simulink model "FOC"  (R2023b)
settings: Solver=FixedStepAuto  StartTime=0.0  StopTime=10.0  FixedStep=1e-4  RelTol=1e-3
settings Model: DataDictionary=FOC.sldd  Creator=18575  LastModifiedBy=18575
settings OptimizationCC: DefaultParameterBehavior=Inlined  UseDivisionForNetSlopeComputation=on  GainParamInheritBuiltInType=on  UseFloatMulNetSlope=on  InlineInvariantSignals=on  PassReuseOutputArgsAs=Individual arguments  ZeroExternalMemoryAtStartup=off  ZeroInternalMemoryAtStartup=off  NoFixptDivByZeroProtection=on  EfficientFloat2IntCast=on  LifeSpan=1  OptimizeBlockOrder=speed  DifferentSizesBufferReuse=on  EfficientTunableParamExpr=on
settings DebuggingCC: ParameterTunabilityLossMsg=error
settings HardwareCC: ProdBitPerPointer=32  ProdBitPerSizeT=32  ProdBitPerPtrDiffT=32  ProdLargestAtomicInteger=Long  ProdLargestAtomicFloat=Double  ProdWordSize=32  ProdLongLongMode=on  ProdHWDeviceType=ARM Compatible->ARM Cortex-M
settings SFSimCC: MATLABDynamicMemAlloc=off
settings RTWCC: Description=Embedded Coder  SystemTargetFile=ert.tlc  TemplateMakefile=ert_default_tmf  GenerateReport=on  LaunchReport=on
settings CodeAppCC: ForceParamTrailComments=on  IgnoreCustomStorageClasses=off  OperatorAnnotations=on  SimulinkDataObjDesc=on  SFDataObjDesc=on  CustomSymbolStrGlobalVar=rt$N$M  CustomSymbolStrType=$N$M  CustomSymbolStrFcn=$N$M$F  CustomSymbolStrMacro=$N$M  InsertBlockDesc=on
settings ERTTargetCC: TargetLangStandard=C99 (ISO)  CodeReplacementLibrary=ARM Cortex-M  GenerateSampleERTMain=on  IncludeMdlTerminateFcn=off  CombineSignalStateStructs=on  SuppressErrorStatus=on  SupportAbsoluteTime=off  SupportNonFinite=off  SupportComplex=off  InlinedParameterPlacement=NonHierarchical  ERTCustomFileTemplate=example_file_process.tlc  ERTFilePackagingFormat=CompactWithDataFile

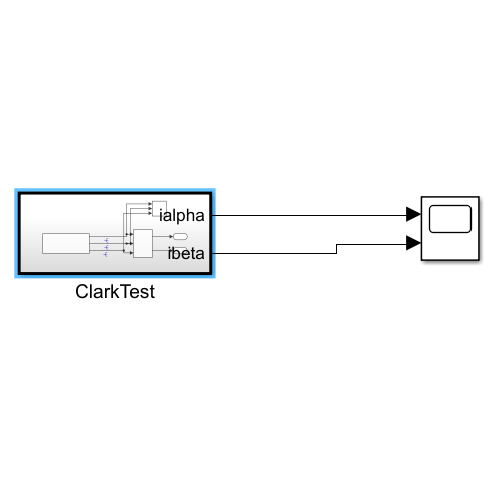
[thumbnail: Simulink's stored preview of the top-level diagram]
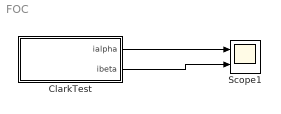
== system FOC ==
  ClarkTest : Subsystem  TreatAsAtomicUnit=on
  Scope1 : Scope  NumInputPorts=2
  wires:
  ClarkTest/1(ialpha) -> Scope1/1
  ClarkTest/2(ibeta) -> Scope1/2

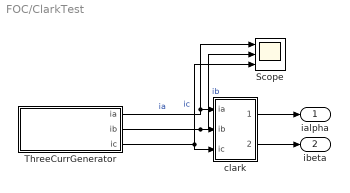
== system FOC/ClarkTest ==
  Scope : Scope  NumInputPorts=3
  ThreeCurrGenerator : Subsystem
  clark : Subsystem
  ialpha : Outport
  ibeta : Outport  Port=2
  wires:
  clark/2(ibeta) -> ibeta/1
  ThreeCurrGenerator/2(ib) -> Scope/2, clark/2(ib)  "ib"
  ThreeCurrGenerator/1(ia) -> Scope/1, clark/1(ia)  "ia"
  ThreeCurrGenerator/3(ic) -> clark/3(ic), Scope/3  "ic"
  clark/1(ialpha) -> ialpha/1

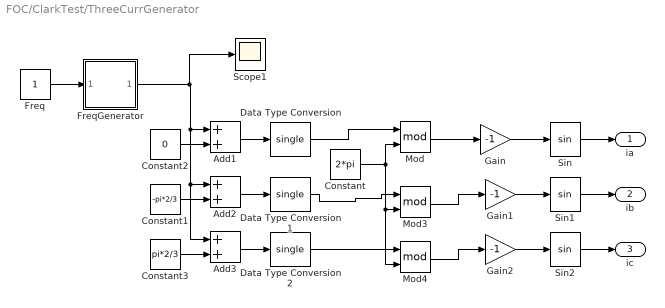
== system FOC/ClarkTest/ThreeCurrGenerator ==
  Add1 : Sum  OutDataTypeStr=single  AccumDataTypeStr=single
  Add2 : Sum  OutDataTypeStr=single  AccumDataTypeStr=single
  Add3 : Sum  OutDataTypeStr=single  AccumDataTypeStr=single
  Constant : Constant  Value=2*pi  OutDataTypeStr=single
  Constant1 : Constant  Value=-pi*2/3  OutDataTypeStr=single
  Constant2 : Constant  Value=0  OutDataTypeStr=single
  Constant3 : Constant  Value=pi*2/3  OutDataTypeStr=single
  Data Type Conversion : DataTypeConversion  OutDataTypeStr=single  SaturateOnIntegerOverflow=off  RndMeth=Floor
  Data Type Conversion1 : DataTypeConversion  OutDataTypeStr=single  SaturateOnIntegerOverflow=off  RndMeth=Floor
  Data Type Conversion2 : DataTypeConversion  OutDataTypeStr=single  SaturateOnIntegerOverflow=off  RndMeth=Floor
  Freq : Constant  OutDataTypeStr=single
  FreqGenerator : Subsystem
  Gain : Gain  Gain=-1
  Gain1 : Gain  Gain=-1
  Gain2 : Gain  Gain=-1
  Mod : Math  Operator=mod
  Mod3 : Math  Operator=mod
  Mod4 : Math  Operator=mod
  Scope1 : Scope
  Sin : Trigonometry  ApproximationMethod=Lookup
  Sin1 : Trigonometry  ApproximationMethod=Lookup
  Sin2 : Trigonometry  ApproximationMethod=Lookup
  ia : Outport
  ib : Outport  Port=2
  ic : Outport  Port=3
  wires:
  Gain1/1 -> Sin1/1
  FreqGenerator/1(Theta) -> Scope1/1, Add3/1, Add2/1, Add1/1
  Add1/1 -> Data Type Conversion/1
  Constant3/1 -> Add3/2
  Add2/1 -> Data Type Conversion1/1
  Constant2/1 -> Add1/2
  Freq/1 -> FreqGenerator/1(Freq)
  Gain2/1 -> Sin2/1
  Constant1/1 -> Add2/2
  Data Type Conversion2/1 -> Mod4/1
  Sin1/1 -> ib/1
  Data Type Conversion/1 -> Mod/1
  Gain/1 -> Sin/1
  Sin/1 -> ia/1
  Mod3/1 -> Gain1/1
  Mod/1 -> Gain/1
  Add3/1 -> Data Type Conversion2/1
  Data Type Conversion1/1 -> Mod3/1
  Sin2/1 -> ic/1
  Constant/1 -> Mod4/2, Mod3/2, Mod/2
  Mod4/1 -> Gain2/1

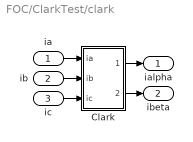
== system FOC/ClarkTest/clark ==
  ia : Inport
  ib : Inport  Port=2
  ic : Inport  Port=3
  Clark : Subsystem
  ialpha : Outport
  ibeta : Outport  Port=2
  wires:
  ia/1 -> Clark/1(ia)
  ib/1 -> Clark/2(ib)
  ic/1 -> Clark/3(ic)
  Clark/1(ialpha) -> ialpha/1
  Clark/2(ibeta) -> ibeta/1

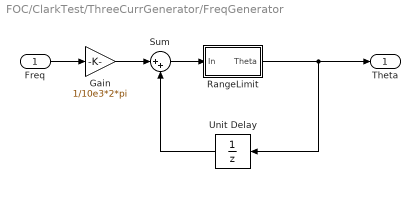
== system FOC/ClarkTest/ThreeCurrGenerator/FreqGenerator ==
  Freq : Inport
  Gain : Gain  Gain=1/10e3*2*pi  OutDataTypeStr=single
  RangeLimit : Subsystem
  Sum : Sum  Inputs=|++  OutDataTypeStr=Inherit: Same as first input
  Unit Delay : UnitDelay  SampleTime=-1  HasFrameUpgradeWarning=on
  Theta : Outport
  wires:
  Freq/1 -> Gain/1
  RangeLimit/1(Theta) -> Theta/1, Unit Delay/1
  Gain/1 -> Sum/1
  Sum/1 -> RangeLimit/1(In)
  Unit Delay/1 -> Sum/2

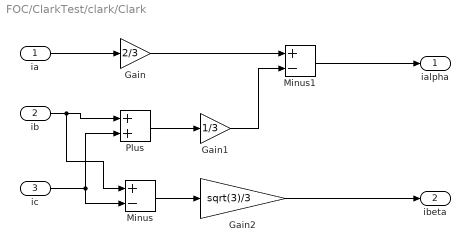
== system FOC/ClarkTest/clark/Clark ==
  ia : Inport
  ib : Inport  Port=2
  ic : Inport  Port=3
  Gain : Gain  Gain=2/3
  Gain1 : Gain  Gain=1/3
  Gain2 : Gain  Gain=sqrt(3)/3
  Minus : Sum  Inputs=+-
  Minus1 : Sum  Inputs=+-
  Plus : Sum
  ialpha : Outport
  ibeta : Outport  Port=2
  wires:
  Gain/1 -> Minus1/1
  Plus/1 -> Gain1/1
  ic/1 -> Minus/2, Plus/2
  Gain1/1 -> Minus1/2
  Gain2/1 -> ibeta/1
  Minus1/1 -> ialpha/1
  ia/1 -> Gain/1
  Minus/1 -> Gain2/1
  ib/1 -> Minus/1, Plus/1

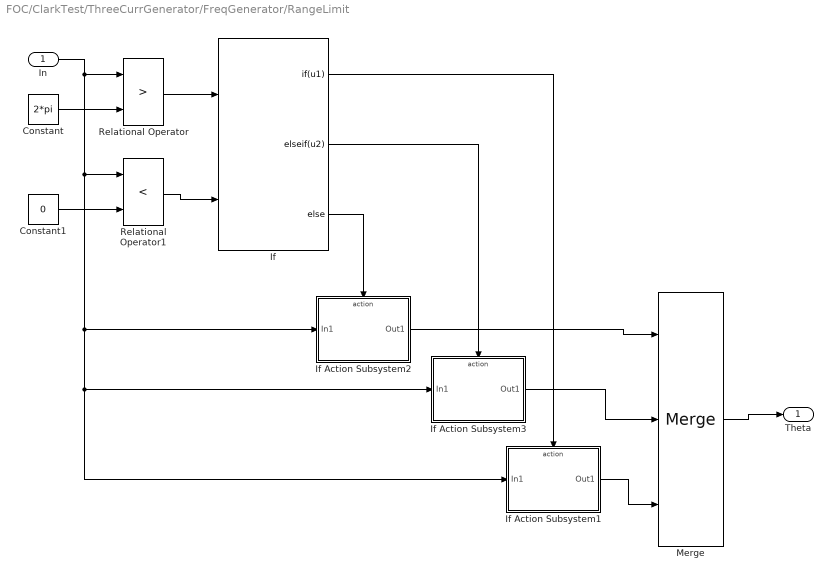
== system FOC/ClarkTest/ThreeCurrGenerator/FreqGenerator/RangeLimit ==
  In : Inport
  Constant : Constant  Value=2*pi  OutDataTypeStr=single  SampleTime=-1
  Constant1 : Constant  Value=0  OutDataTypeStr=single  SampleTime=-1
  If : If  NumInputs=2  IfExpression=u1  ElseIfExpressions=u2
  If Action Subsystem1 : Subsystem  TreatAsAtomicUnit=on
  If Action Subsystem2 : Subsystem  TreatAsAtomicUnit=on
  If Action Subsystem3 : Subsystem  TreatAsAtomicUnit=on
  Merge : Merge  Inputs=3
  Relational Operator : RelationalOperator  Operator=>  OutDataTypeStr=boolean  RndMeth=Simplest  InputSameDT=off
  Relational Operator1 : RelationalOperator  Operator=<  OutDataTypeStr=boolean  RndMeth=Simplest  InputSameDT=off
  Theta : Outport
  wires:
  Relational Operator/1 -> If/1
  Constant/1 -> Relational Operator/2
  In/1 -> Relational Operator1/1, If Action Subsystem2/1(In1), If Action Subsystem3/1(In1), If Action Subsystem1/1(In1), Relational Operator/1
  Merge/1 -> Theta/1
  If/3 -> If Action Subsystem2/Action
  If/1 -> If Action Subsystem1/Action
  If Action Subsystem2/1(Out1) -> Merge/1
  Constant1/1 -> Relational Operator1/2
  Relational Operator1/1 -> If/2
  If/2 -> If Action Subsystem3/Action
  If Action Subsystem1/1(Out1) -> Merge/3
  If Action Subsystem3/1(Out1) -> Merge/2

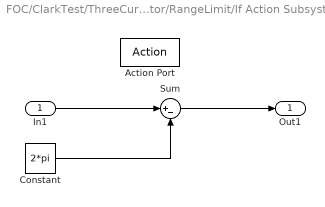
== system FOC/ClarkTest/ThreeCurrGenerator/FreqGenerator/RangeLimit/If Action Subsystem1 ==
  In1 : Inport
  Action Port : ActionPort  ActionPortLabel=if(u1)
  Constant : Constant  Value=2*pi  OutDataTypeStr=single  SampleTime=-1
  Sum : Sum  Inputs=|+-
  Out1 : Outport
  wires:
  In1/1 -> Sum/1
  Constant/1 -> Sum/2
  Sum/1 -> Out1/1

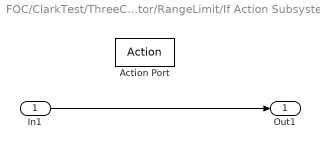
== system FOC/ClarkTest/ThreeCurrGenerator/FreqGenerator/RangeLimit/If Action Subsystem2 ==
  In1 : Inport
  Action Port : ActionPort  ActionPortLabel=else
  Out1 : Outport
  wires:
  In1/1 -> Out1/1

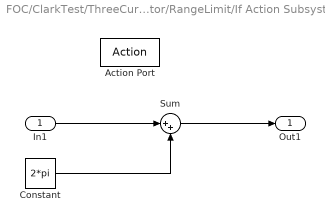
== system FOC/ClarkTest/ThreeCurrGenerator/FreqGenerator/RangeLimit/If Action Subsystem3 ==
  In1 : Inport
  Action Port : ActionPort  ActionPortLabel=elseif(u2)
  Constant : Constant  Value=2*pi  OutDataTypeStr=single  SampleTime=-1
  Sum : Sum  Inputs=|++
  Out1 : Outport
  wires:
  Constant/1 -> Sum/2
  In1/1 -> Sum/1
  Sum/1 -> Out1/1
